simulink library "Enrg_conv_El_to_Mec_Bosch"  (R2016a)
settings: Solver=ode1  StartTime=0.0  StopTime=Inf  FixedStep=0.001  RelTol=1e-3
undefined symbols (not defined in the file): drvEmot_RefTqeMOT, FirstDrivenAxle_FirstDrivenAxleNoOfEmot, FMIKit, SecondDrivenAxle_SecondDrivenAxleNoOfEmot
libraries: Enrg_conv_El_to_Mec_Bosch x13, Electrical_converter x8
(part 1 of 5)
settings Model: Creator=SAHOPRA  LastModifiedBy=fschmi1
settings DataIOCC: LimitDataPoints=on  SaveFormat=Array
settings OptimizationCC: BlockReduction=off  OptimizeBlockIOStorage=off  BufferReuse=off  GlobalBufferReuse=off  ExpressionFolding=off  ExpressionDepthLimit=2147483647  LocalBlockOutputs=off
settings DebuggingCC: UnderspecifiedInitializationDetection=Classic  MergeDetectMultiDrivingBlocksExec=none  SolverPrmCheckMsg=warning  StateNameClashWarn=warning
settings HardwareCC: ProdBitPerPointer=32  ProdLargestAtomicFloat=None  ProdIntDivRoundTo=Undefined  ProdEndianess=Unspecified  ProdWordSize=32  ProdHWDeviceType=32-bit Generic
settings ModelReferenceCC: PropagateSignalLabelsOutOfModel=off
settings SFSimCC: SimUserSources="\"C:\\ORNOVNU\\01_DIVe\\drl_dev_hvlv_work\\ldDevProj\\case\\c000\\Content\\phys\\hvs\\Support\\FMIToolkit\\FMIKit-Simulink-2.9\\src\\FMU.cpp\" \"C:\\ORNOVNU\\01_DIVe\\drl_dev_hvlv_work\\ldDevProj\\case\\c000\\Content\\phys\\hvs\\Support\\FMIToolkit\\FMIKit-Simulink-2.9\\src\\FMU1.cpp\" \"C:\\ORNOVNU\\01_DIVe\\drl_dev_hvlv_work\\ldDevProj\\case\\c000\\Content\\phys\\hvs\\Support\\FMIToolkit\\FMIKit-Simulink-2.9\\src\\FMU2.cpp\" \"C:\\ORNOVNU\\01_DIVe\\drm_dev_hvlv_work\\Content\\phys\\hvs\\Support\\FMIToolkit\\FMIKit-Simulink-2.9\\src\\FMU.cpp\" \"C:\\ORNOVNU\\01_DIVe\\drm_dev_hvlv_work\\Content\\phys\\hvs\\Support\\FMIToolkit\\FMIKit-Simulink-2.9\\src\\FMU1.cpp\" \"C:\\ORNOVNU\\01_DIVe\\drm_dev_hvlv_work\\Content\\phys\\hvs\\Support\\FMIToolkit\\FMIKit-Simulink-2.9\\src\\FMU2.cpp\" \"C:\\ORNOVNU\\01_DIVe\\drm_dev_hvlv_work\\Content\\phys\\hvs\\detailed\\Support\\FMIToolkit\\FMIKit-Simulink-2.9\\src\\FMU.cpp\" \"C:\\ORNOVNU\\01_DIVe\\drm_dev_hvlv_work\\Content\\phys\\hvs\\detailed\\Support\\FMIToolkit\\FMIKit-Simulink-2.9\\src\\FMU1.cpp\" \"C:\\ORNOVNU\\01_DIVe\\drm_dev_hvlv_work\\Content\\phys\\hvs\\detailed\\Support\\FMIToolkit\\FMIKit-Simulink-2.9\\src\\FMU2.cpp\" \"Y:\\03_Tasks\\20210223_OrNu_HVSDive_BoschModelle\\02_WIP\\FMIKit-Simulink-2.9\\src\\FMU.cpp\" \"Y:\\03_Tasks\\20210223_OrNu_HVSDive_BoschModelle\\02_WIP\\FMIKit-Simulink-2.9\\src\\FMU1.cpp\" \"Y:\\03_Tasks\\20210223_OrNu_HVSDive_BoschModelle\\02_WIP\\FMIKit-Simulink-2.9\\src\\FMU2.cpp\" \"T:\\DIVe\\drm_dev_hvlv_work\\Content\\phys\\hvs\\detailed\\Support\\FMIToolkit\\FMIKit-Simulink-2.9\\src\\FMU.cpp\" \"T:\\DIVe\\drm_dev_hvlv_work\\Content\\phys\\hvs\\detailed\\Support\\FMIToolkit\\FMIKit-Simulink-2.9\\src\\FMU1.cpp\" \"T:\\DIVe\\drm_dev_hvlv_work\\Content\\phys\\hvs\\detailed\\Support\\FMIToolkit\\FMIKit-Simulink-2.9\\src\\FMU2.cpp\" \"c:\\ORNOVNU\\01_DIVe\\drm_dev_hvlv_work\\Content\\phys\\hvs\\detailed\\Support\\FMIToolkit\\FMIKit-Simulink-2.9\\src\\FMU.cpp\" \"c:\\ORNOVNU\\01_DIVe\\drm_dev_hvlv_work\\Content\\phys\\hvs\\detailed\\Support\\FMIToolkit\\FMIKit-Simulink-2.9\\src\\FMU1.cpp\" \"c:\\ORNOVNU\\01_DIVe\\drm_dev_hvlv_work\\Content\\phys\\hvs\\detailed\\Support\\FMIToolkit\\FMIKit-Simulink-2.9\\src\\FMU2.cpp\" \"D:\\01_DIVe\\drm_dev_hvlv_work\\Content\\phys\\hvs\\detailed\\Support\\FMIToolkit\\FMIKit-Simulink-2.9\\src\\FMU.cpp\" \"D:\\01_DIVe\\drm_dev_hvlv_work\\Content\\phys\\hvs\\detailed\\Support\\FMIToolkit\\FMIKit-Simulink-2.9\\src\\FMU1.cpp\" \"D:\\01_DIVe\\drm_dev_hvlv_work\\Content\\phys\\hvs\\detailed\\Support\\FMIToolkit\\FMIKit-Simulink-2.9\\src\\FMU2.cpp\" \"D:\\DIVe_Streams\\drm_dev_hvlv_work_1098\\Content\\phys\\hvs\\detailed\\Support\\FMIToolkit\\FMIKit-Simulink-2.9\\src\\FMU.cpp\" \"D:\\DIVe_Streams\\drm_dev_hvlv_work_1098\\Content\\phys\\hvs\\detailed\\Support\\FMIToolkit\\FMIKit-Simulink-2.9\\src\\FMU1.cpp\" \"D:\\DIVe_Streams\\drm_dev_hvlv_work_1098\\Content\\phys\\hvs\\detailed\\Support\\FMIToolkit\\FMIKit-Simulink-2.9\\src\\FMU2.cpp\""  SimUserIncludeDirs="\"C:\\ORNOVNU\\01_DIVe\\drl_dev_hvlv_work\\ldDevProj\\case\\c000\\Content\\phys\\hvs\\Support\\FMIToolkit\\FMIKit-Simulink-2.9\\include\" \"C:\\ORNOVNU\\01_DIVe\\drm_dev_hvlv_work\\Content\\phys\\hvs\\Support\\FMIToolkit\\FMIKit-Simulink-2.9\\include\" \"C:\\ORNOVNU\\01_DIVe\\drm_dev_hvlv_work\\Content\\phys\\hvs\\detailed\\Support\\FMIToolkit\\FMIKit-Simulink-2.9\\include\" \"Y:\\03_Tasks\\20210223_OrNu_HVSDive_BoschModelle\\02_WIP\\FMIKit-Simulink-2.9\\include\" \"T:\\DIVe\\drm_dev_hvlv_work\\Content\\phys\\hvs\\detailed\\Support\\FMIToolkit\\FMIKit-Simulink-2.9\\include\" \"c:\\ORNOVNU\\01_DIVe\\drm_dev_hvlv_work\\Content\\phys\\hvs\\detailed\\Support\\FMIToolkit\\FMIKit-Simulink-2.9\\include\" \"D:\\01_DIVe\\drm_dev_hvlv_work\\Content\\phys\\hvs\\detailed\\Support\\FMIToolkit\\FMIKit-Simulink-2.9\\include\" \"D:\\DIVe_Streams\\drm_dev_hvlv_work_1098\\Content\\phys\\hvs\\detailed\\Support\\FMIToolkit\\FMIKit-Simulink-2.9\\include\""
settings RTWCC: SystemTargetFile=rti1005.tlc  MakeCommand=make_rti  TemplateMakefile=rti1005.tmf  Description=dSPACE DS1005 Hardware Platform  CustomInclude="\"C:\\ORNOVNU\\01_DIVe\\drl_dev_hvlv_work\\ldDevProj\\case\\c000\\Content\\phys\\hvs\\Support\\FMIToolkit\\FMIKit-Simulink-2.9\\include\" \"C:\\ORNOVNU\\01_DIVe\\drm_dev_hvlv_work\\Content\\phys\\hvs\\Support\\FMIToolkit\\FMIKit-Simulink-2.9\\include\" \"C:\\ORNOVNU\\01_DIVe\\drm_dev_hvlv_work\\Content\\phys\\hvs\\detailed\\Support\\FMIToolkit\\FMIKit-Simulink-2.9\\include\" \"Y:\\03_Tasks\\20210223_OrNu_HVSDive_BoschModelle\\02_WIP\\FMIKit-Simulink-2.9\\include\" \"T:\\DIVe\\drm_dev_hvlv_work\\Content\\phys\\hvs\\detailed\\Support\\FMIToolkit\\FMIKit-Simulink-2.9\\include\" \"c:\\ORNOVNU\\01_DIVe\\drm_dev_hvlv_work\\Content\\phys\\hvs\\detailed\\Support\\FMIToolkit\\FMIKit-Simulink-2.9\\include\" \"D:\\01_DIVe\\drm_dev_hvlv_work\\Content\\phys\\hvs\\detailed\\Support\\FMIToolkit\\FMIKit-Simulink-2.9\\include\" \"D:\\DIVe_Streams\\drm_dev_hvlv_work_1098\\Content\\phys\\hvs\\detailed\\Support\\FMIToolkit\\FMIKit-Simulink-2.9\\include\""  CustomSource="\"C:\\ORNOVNU\\01_DIVe\\drl_dev_hvlv_work\\ldDevProj\\case\\c000\\Content\\phys\\hvs\\Support\\FMIToolkit\\FMIKit-Simulink-2.9\\src\\FMU.cpp\" \"C:\\ORNOVNU\\01_DIVe\\drl_dev_hvlv_work\\ldDevProj\\case\\c000\\Content\\phys\\hvs\\Support\\FMIToolkit\\FMIKit-Simulink-2.9\\src\\FMU1.cpp\" \"C:\\ORNOVNU\\01_DIVe\\drl_dev_hvlv_work\\ldDevProj\\case\\c000\\Content\\phys\\hvs\\Support\\FMIToolkit\\FMIKit-Simulink-2.9\\src\\FMU2.cpp\" \"C:\\ORNOVNU\\01_DIVe\\drm_dev_hvlv_work\\Content\\phys\\hvs\\Support\\FMIToolkit\\FMIKit-Simulink-2.9\\src\\FMU.cpp\" \"C:\\ORNOVNU\\01_DIVe\\drm_dev_hvlv_work\\Content\\phys\\hvs\\Support\\FMIToolkit\\FMIKit-Simulink-2.9\\src\\FMU1.cpp\" \"C:\\ORNOVNU\\01_DIVe\\drm_dev_hvlv_work\\Content\\phys\\hvs\\Support\\FMIToolkit\\FMIKit-Simulink-2.9\\src\\FMU2.cpp\" \"C:\\ORNOVNU\\01_DIVe\\drm_dev_hvlv_work\\Content\\phys\\hvs\\detailed\\Support\\FMIToolkit\\FMIKit-Simulink-2.9\\src\\FMU.cpp\" \"C:\\ORNOVNU\\01_DIVe\\drm_dev_hvlv_work\\Content\\phys\\hvs\\detailed\\Support\\FMIToolkit\\FMIKit-Simulink-2.9\\src\\FMU1.cpp\" \"C:\\ORNOVNU\\01_DIVe\\drm_dev_hvlv_work\\Content\\phys\\hvs\\detailed\\Support\\FMIToolkit\\FMIKit-Simulink-2.9\\src\\FMU2.cpp\" \"Y:\\03_Tasks\\20210223_OrNu_HVSDive_BoschModelle\\02_WIP\\FMIKit-Simulink-2.9\\src\\FMU.cpp\" \"Y:\\03_Tasks\\20210223_OrNu_HVSDive_BoschModelle\\02_WIP\\FMIKit-Simulink-2.9\\src\\FMU1.cpp\" \"Y:\\03_Tasks\\20210223_OrNu_HVSDive_BoschModelle\\02_WIP\\FMIKit-Simulink-2.9\\src\\FMU2.cpp\" \"T:\\DIVe\\drm_dev_hvlv_work\\Content\\phys\\hvs\\detailed\\Support\\FMIToolkit\\FMIKit-Simulink-2.9\\src\\FMU.cpp\" \"T:\\DIVe\\drm_dev_hvlv_work\\Content\\phys\\hvs\\detailed\\Support\\FMIToolkit\\FMIKit-Simulink-2.9\\src\\FMU1.cpp\" \"T:\\DIVe\\drm_dev_hvlv_work\\Content\\phys\\hvs\\detailed\\Support\\FMIToolkit\\FMIKit-Simulink-2.9\\src\\FMU2.cpp\" \"c:\\ORNOVNU\\01_DIVe\\drm_dev_hvlv_work\\Content\\phys\\hvs\\detailed\\Support\\FMIToolkit\\FMIKit-Simulink-2.9\\src\\FMU.cpp\" \"c:\\ORNOVNU\\01_DIVe\\drm_dev_hvlv_work\\Content\\phys\\hvs\\detailed\\Support\\FMIToolkit\\FMIKit-Simulink-2.9\\src\\FMU1.cpp\" \"c:\\ORNOVNU\\01_DIVe\\drm_dev_hvlv_work\\Content\\phys\\hvs\\detailed\\Support\\FMIToolkit\\FMIKit-Simulink-2.9\\src\\FMU2.cpp\" \"D:\\01_DIVe\\drm_dev_hvlv_work\\Content\\phys\\hvs\\detailed\\Support\\FMIToolkit\\FMIKit-Simulink-2.9\\src\\FMU.cpp\" \"D:\\01_DIVe\\drm_dev_hvlv_work\\Content\\phys\\hvs\\detailed\\Support\\FMIToolkit\\FMIKit-Simulink-2.9\\src\\FMU1.cpp\" \"D:\\01_DIVe\\drm_dev_hvlv_work\\Content\\phys\\hvs\\detailed\\Support\\FMIToolkit\\FMIKit-Simulink-2.9\\src\\FMU2.cpp\" \"D:\\DIVe_Streams\\drm_dev_hvlv_work_1098\\Content\\phys\\hvs\\detailed\\Support\\FMIToolkit\\FMIKit-Simulink-2.9\\src\\FMU.cpp\" \"D:\\DIVe_Streams\\drm_dev_hvlv_work_1098\\Content\\phys\\hvs\\detailed\\Support\\FMIToolkit\\FMIKit-Simulink-2.9\\src\\FMU1.cpp\" \"D:\\DIVe_Streams\\drm_dev_hvlv_work_1098\\Content\\phys\\hvs\\detailed\\Support\\FMIToolkit\\FMIKit-Simulink-2.9\\src\\FMU2.cpp\""
settings STFCustomTargetCC: ModelReferenceCompliant=off  GeneratePreprocessorConditionals=Disable all  CombineOutputUpdateFcns=on  MatFileLogging=on  CPPClassGenCompliant=on  GRTInterface=off  SystemTargetFile=rti1005.tlc
settings GRTTargetCC: ModelReferenceCompliant=off  ParMdlRefBuildCompliant=off  CompOptLevelCompliant=off  ConcurrentExecutionCompliant=off  UseToolchainInfoCompliant=off
settings ConfigComp: CovModelRefEnable=Off

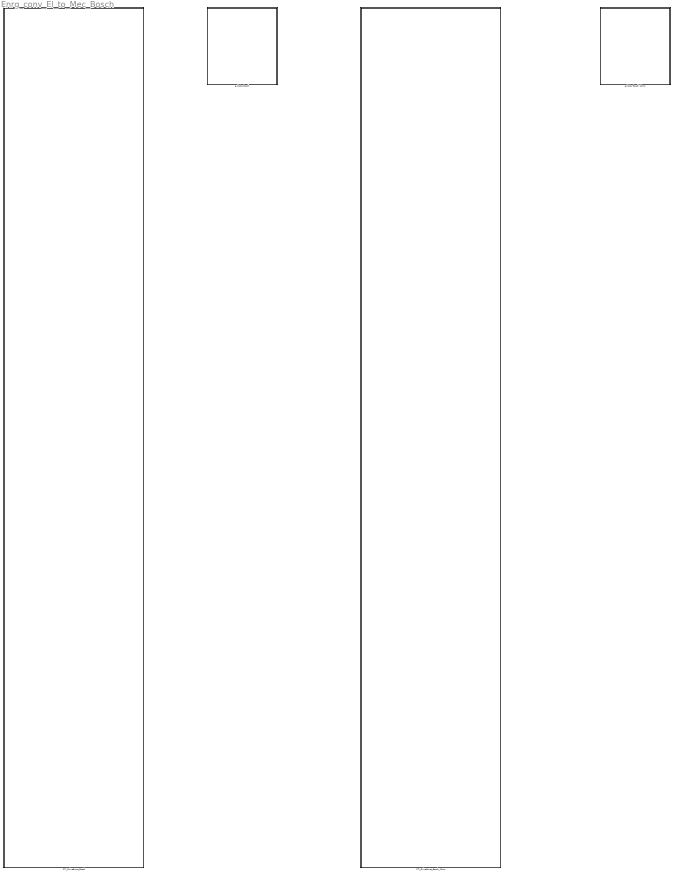
== system Enrg_conv_El_to_Mec_Bosch ==
  PTI_DriveEmot_Bosch : Subsystem  TreatAsAtomicUnit=on  SystemSampleTime=0.1
  PTI_DriveEmot_Bosch_10ms : Subsystem  TreatAsAtomicUnit=on  SystemSampleTime=0.01
  e-Motor Bosch : Subsystem  mask(MapModule){}
  e-Motor Bosch 10ms : Subsystem  mask(MapModule){}

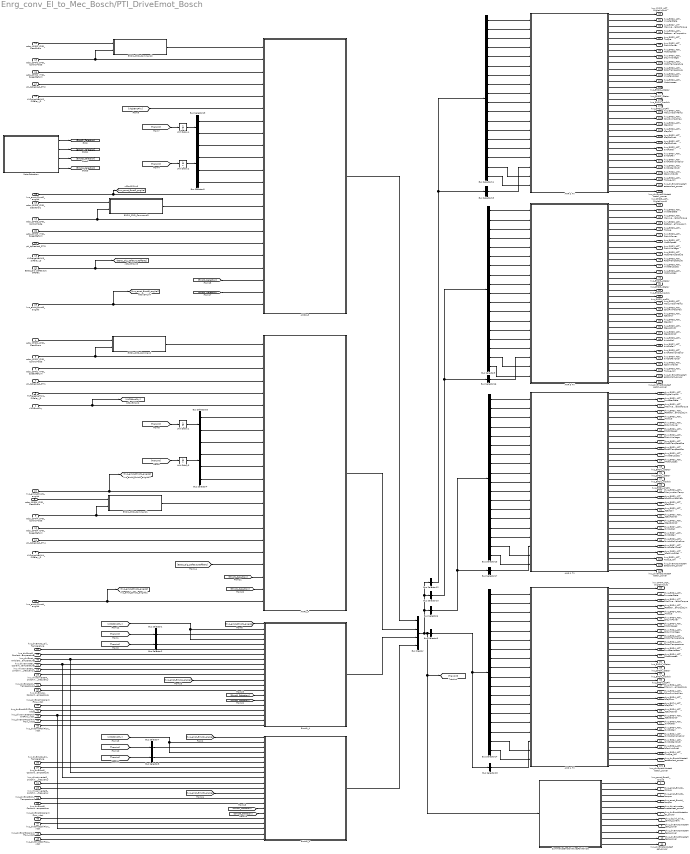
== system Enrg_conv_El_to_Mec_Bosch/PTI_DriveEmot_Bosch ==
  vltZkBmsPhy : Inport
  HVFreigabeHW1_SiRelay_D : Inport  Port=2
  HVFreigabeHW4_SiRelay_D : Inport  Port=3
  edcu_EMD1_CMD_ClearErrors : Inport  Port=4
  edcu_EMD1_CMD_ControlMode : Inport  Port=5
  edcu_EMD1_CMD_SpeedRefLim : Inport  Port=6
  pti_tqDesired_PTI1 : Inport  Description=[Nm]  Port=7
      settings: AttributesFormatString=%<Description>
  edcu_EMD4_CMD_ClearErrors : Inport  Port=8
  edcu_EMD4_CMD_ControlMode : Inport  Port=9
  edcu_EMD4_CMD_SpeedRefLim : Inport  Port=10
  pti_tqDesired_PTI4 : Inport  Description=[Nm]  Port=11
      settings: AttributesFormatString=%<Description>
  HVFreigabeHW2_SiRelay_D : Inport  Port=12
  HVFreigabeHW3_SiRelay_D : Inport  Port=13
  edcu_EMD2_CMD_ClearErrors : Inport  Port=14
  edcu_EMD2_CMD_ControlMode : Inport  Port=15
  edcu_EMD2_CMD_SpeedRefLim : Inport  Port=16
  pti_tqDesired_PTI2 : Inport  Description=[Nm]  Port=17
      settings: AttributesFormatString=%<Description>
  edcu_EMD3_CMD_ClearErrors : Inport  Port=18
  edcu_EMD3_CMD_ControlMode : Inport  Port=19
  edcu_EMD3_CMD_SpeedRefLim : Inport  Port=20
  pti_tqDesired_PTI3 : Inport  Description=[Nm]  Port=21
      settings: AttributesFormatString=%<Description>
  EDCU_Dig_SafetyCutOffDG1 : Inport  Port=22
  hvs_driveInverter1_switching_frequency : Inport  Port=23
  hvs_driveInverter2_switching_frequency : Inport  Port=24
  hvs_driveInverter3_switching_frequency : Inport  Port=25
  hvs_driveInverter4_switching_frequency : Inport  Port=26
  hvs_emot_Emot1_angVel : Inport  Port=27
  hvs_emot_Emot2_angVel : Inport  Port=28
  hvs_emot_Emot3_angVel : Inport  Port=29
  hvs_emot_Emot4_angVel : Inport  Port=30
  hvs_driveInverter_coolant_temperature : Inport  Port=31
  hvs_drvEmot1_Oil_Temperature : Inport  Port=32
  hvs_drvEmot1_Coolant_Temperature : Inport  Port=33
  hvs_drvEmot4Oil_Temperature : Inport  Port=34
  hvs_drvEmot4_Coolant_Temperature : Inport  Port=35
  hvs_drvEmot2_Oil_Temperature : Inport  Port=36
  hvs_drvEmot2_Coolant_Temperature : Inport  Port=37
  hvs_drvEmot3Oil_Temperature : Inport  Port=38
  hvs_drvEmot3_Coolant_Temperature : Inport  Port=39
  hvs_drvEmot_Ambient_Temperature : Inport  Port=40
  hvs_drvEmot1CoolantFlow_vdot : Inport  Port=41
  hvs_drvEmot1OilFlow_vdot : Inport  Port=42
  hvs_driveInverterCoolantFlow_vdot : Inport  Port=43
  hvs_drvEmot4CoolantFlow_vdot : Inport  Port=44
  hvs_drvEmot4OilFlow_vdot : Inport  Port=45
  hvs_drvEmot2CoolantFlow_vdot : Inport  Port=46
  hvs_drvEmot2OilFlow_vdot : Inport  Port=47
  hvs_drvEmot3CoolantFlow_vdot : Inport  Port=48
  hvs_drvEmot3OilFlow_vdot : Inport  Port=49
  AWR 1 TX : Subsystem
  AWR 2 TX : Subsystem
  AWR 3 TX : Subsystem
  AWR 4 TX : Subsystem
  AWR1_4 : Subsystem
  AWR2_3 : Subsystem
  Bus Selector11 : BusSelector  OutputSignals=EMD2_ACT_DcLinkVoltage,EMD_ACT_DigitalInput1,EMD_ACT_MaximumAvailableTorque,EMD_ACT_DcLinkPower,EMD_ACT_MotorSpeed,EMD_ACT_MotorTorque,EMD_ACT_InverterState,EMD_ACT_ReferenceTorqueLimited,drvEmot_T_Stator,drvEmot_T_Rotor,Inv_Ploss,mot_Ploss,uStator,iStator,modIdx,cosPhi,wasteHeat_coolant,wasteHeat_oil
  Bus Selector13 : BusSelector  OutputSignals=EMD1_ACT_DcLinkVoltage,EMD_ACT_DigitalInput1,EMD_ACT_MaximumAvailableTorque,EMD_ACT_DcLinkPower,EMD_ACT_MotorSpeed,EMD_ACT_MotorTorque,EMD_ACT_InverterState,EMD_ACT_ReferenceTorqueLimited,drvEmot_T_Stator,drvEmot_T_Rotor,Inv_Ploss,mot_Ploss,uStator,iStator,modIdx,cosPhi,wasteHeat_coolant,wasteHeat_oil
  Bus Selector14 : BusSelector  OutputSignals=EMD4_ACT_DcLinkVoltage,EMD_ACT_DigitalInput1,EMD_ACT_MaximumAvailableTorque,EMD_ACT_DcLinkPower,EMD_ACT_MotorSpeed,EMD_ACT_MotorTorque,EMD_ACT_InverterState,EMD_ACT_ReferenceTorqueLimited,drvEmot_T_Stator,drvEmot_T_Rotor,Inv_Ploss,mot_Ploss,uStator,iStator,modIdx,cosPhi,wasteHeat_coolant,wasteHeat_oil
  Bus Selector{15..18} (4 alike) : BusSelector  OutputSignals=driveInverter_Temperatures  OutputAsBus=on
  Bus Selector9 : BusSelector  OutputSignals=EMD3_ACT_DcLinkVoltage,EMD_ACT_DigitalInput1,EMD_ACT_MaximumAvailableTorque,EMD_ACT_DcLinkPower,EMD_ACT_MotorSpeed,EMD_ACT_MotorTorque,EMD_ACT_InverterState,EMD_ACT_ReferenceTorqueLimited,drvEmot_T_Stator,drvEmot_T_Rotor,Inv_Ploss,mot_Ploss,uStator,iStator,modIdx,cosPhi,wasteHeat_oil,wasteHeat_coolant
  Bus Creator : BusCreator  Inputs=4
  Bus Selector1 : BusSelector  OutputSignals=awr1_4B.awr1B.trqEmotDesPhy
  Bus Selector10 : BusSelector  OutputSignals=awr2_3B.awr3B.EMD3_ACT_DcLinkVoltage,awr2_3B.awr3B.EMD_ACT_DigitalInput1,awr2_3B.awr3B.EMD_ACT_MaximumAvailableTorque,awr2_3B.awr3B.EMD_ACT_DcLinkPower,awr2_3B.awr3B.EMD_ACT_MotorSpeed,awr2_3B.awr3B.EMD_ACT_MotorTorque,awr2_3B.awr3B.EMD_ACT_InverterState,awr2_3B.awr3B.EMD_ACT_ReferenceTorqueLimited,awr2_3B.awr3B.trqEmotDesPhy,emot2_3B.emot3B.driveInverter_Temperatures,emot2_3B.emot3B.drvEmot_T_Stator,emot2_3B.emot3B.drvEmot_T_Rotor,emot2_3B.emot3B.Inv_Ploss,emot2_3B.emot3B.mot_Ploss,emot2_3B.emot3B.uStator,emot2_3B.emot3B.iStator,emot2_3B.emot3B.modIdx,emot2_3B.emot3B.cosPhi,emot2_3B.emot3B.wasteHeat_coolant,emot2_3B.emot3B.wasteHeat_oil  OutputAsBus=on
  Bus Selector12 : BusSelector  OutputSignals=awr2_3B.awr2B.EMD2_ACT_DcLinkVoltage,awr2_3B.awr2B.EMD_ACT_DigitalInput1,awr2_3B.awr2B.EMD_ACT_MaximumAvailableTorque,awr2_3B.awr2B.EMD_ACT_DcLinkPower,awr2_3B.awr2B.EMD_ACT_MotorSpeed,awr2_3B.awr2B.EMD_ACT_MotorTorque,awr2_3B.awr2B.EMD_ACT_InverterState,awr2_3B.awr2B.EMD_ACT_ReferenceTorqueLimited,awr2_3B.awr2B.trqEmotDesPhy,emot2_3B.emot2B.driveInverter_Temperatures,emot2_3B.emot2B.drvEmot_T_Stator,emot2_3B.emot2B.drvEmot_T_Rotor,emot2_3B.emot2B.Inv_Ploss,emot2_3B.emot2B.mot_Ploss,emot2_3B.emot2B.uStator,emot2_3B.emot2B.iStator,emot2_3B.emot2B.modIdx,emot2_3B.emot2B.cosPhi,emot2_3B.emot2B.wasteHeat_coolant,emot2_3B.emot2B.wasteHeat_oil  OutputAsBus=on
  Bus Selector19 : BusSelector  OutputSignals=emot2_3B.emot2B.trqEmotPhy,emot2_3B.emot3B.trqEmotPhy
  Bus Selector2 : BusSelector  OutputSignals=awr1_4B.awr4B.trqEmotDesPhy
  Bus Selector20 : BusSelector  OutputSignals=emot1_4B.emot1B.trqEmotPhy,emot1_4B.emot4B.trqEmotPhy
  Bus Selector3 : BusSelector  OutputSignals=emot2_3B.emot2B.pwrEmotPhy,emot2_3B.emot3B.pwrEmotPhy,emot2_3B.emot2B.trqEmotMax,emot2_3B.emot3B.trqEmotMax
  Bus Selector4 : BusSelector  OutputSignals=emot1_4B.emot1B.pwrEmotPhy,emot1_4B.emot4B.pwrEmotPhy,emot1_4B.emot1B.trqEmotMax,emot1_4B.emot4B.trqEmotMax
  Bus Selector5 : BusSelector  OutputSignals=awr1_4B.awr4B.EMD4_ACT_DcLinkVoltage,awr1_4B.awr4B.EMD_ACT_DigitalInput1,awr1_4B.awr4B.EMD_ACT_MaximumAvailableTorque,awr1_4B.awr4B.EMD_ACT_DcLinkPower,awr1_4B.awr4B.EMD_ACT_MotorSpeed,awr1_4B.awr4B.EMD_ACT_MotorTorque,awr1_4B.awr4B.EMD_ACT_InverterState,awr1_4B.awr4B.EMD_ACT_ReferenceTorqueLimited,awr1_4B.awr4B.trqEmotDesPhy,emot1_4B.emot4B.driveInverter_Temperatures,emot1_4B.emot4B.drvEmot_T_Stator,emot1_4B.emot4B.drvEmot_T_Rotor,emot1_4B.emot4B.Inv_Ploss,emot1_4B.emot4B.mot_Ploss,emot1_4B.emot4B.uStator,emot1_4B.emot4B.iStator,emot1_4B.emot4B.modIdx,emot1_4B.emot4B.cosPhi,emot1_4B.emot4B.wasteHeat_coolant,emot1_4B.emot4B.wasteHeat_oil  OutputAsBus=on
  Bus Selector6 : BusSelector  OutputSignals=awr1_4B.awr1B.EMD1_ACT_DcLinkVoltage,awr1_4B.awr1B.EMD_ACT_DigitalInput1,awr1_4B.awr1B.EMD_ACT_MaximumAvailableTorque,awr1_4B.awr1B.EMD_ACT_DcLinkPower,awr1_4B.awr1B.EMD_ACT_MotorSpeed,awr1_4B.awr1B.EMD_ACT_MotorTorque,awr1_4B.awr1B.EMD_ACT_InverterState,awr1_4B.awr1B.EMD_ACT_ReferenceTorqueLimited,awr1_4B.awr1B.trqEmotDesPhy,emot1_4B.emot1B.driveInverter_Temperatures,emot1_4B.emot1B.drvEmot_T_Stator,emot1_4B.emot1B.drvEmot_T_Rotor,emot1_4B.emot1B.Inv_Ploss,emot1_4B.emot1B.mot_Ploss,emot1_4B.emot1B.uStator,emot1_4B.emot1B.iStator,emot1_4B.emot1B.modIdx,emot1_4B.emot1B.cosPhi,emot1_4B.emot1B.wasteHeat_coolant,emot1_4B.emot1B.wasteHeat_oil  OutputAsBus=on
  Bus Selector7 : BusSelector  OutputSignals=awr2_3B.awr2B.trqEmotDesPhy
  Bus Selector8 : BusSelector  OutputSignals=awr2_3B.awr3B.trqEmotDesPhy
  EMD1_CMD_Command : Subsystem
  EMD1_CMD_Command1 : Subsystem
  EMD1_CMD_Command2 : Subsystem
  EMD1_CMD_Command3 : Subsystem
  Emot1_4 : Subsystem
  Emot2_3 : Subsystem
  MotorSelection : Subsystem
  SummarizeEmotorValuesForVehicle : Subsystem  TreatAsAtomicUnit=on
  Unit Delay{1..4} (4 alike) : UnitDelay  SampleTime=-1
  hvs_dcLink_drive_emot_current : Outport
  hvs_emot_Emot1_torque : Outport  Port=2
  hvs_emot_Emot2_torque : Outport  Port=3
  hvs_emot_Emot3_torque : Outport  Port=4
  hvs_emot_Emot4_torque : Outport  Port=5
  hvs_driveInverter_wasteHeat_power : Outport  Port=6
  hvs_drvEmotWasteHeat_power : Outport  Port=7
  hvs_drvEmot1WasteHeat_power : Outport  Port=8
  hvs_drvEmot2WasteHeat_power : Outport  Port=9
  hvs_drvEmot3WasteHeat_power : Outport  Port=10
  hvs_drvEmot4WasteHeat_power : Outport  Port=11
  hvs_EMD1_ACT_DigitalInput1 : Outport  Port=12
  hvs_EMD1_ACT_InverterState : Outport  Port=13
  hvs_EMD1_ACT_MaxAvailableTorque : Outport  Port=14
  hvs_EMD1_ACT_ReferenceTorqueLim : Outport  Port=15
  hvs_EMD1_ACT_Torque : Outport  Port=16
  hvs_EMD1_ACT_DcLinkPower : Outport  Port=17
  hvs_EMD1_ACT_MotorSpeed : Outport  Port=18
  hvs_EMD1_ACT_DcLinkVoltage : Outport  Port=19
  hvs_EMD1_ACT_MaxJunctionTemp : Outport  Port=20
  hvs_EMD1_ACT_MotorTemperature : Outport  Port=21
  hvs_EMD1_ACT_RotorTemperature : Outport  Port=22
  hvs_EMD1_ACT_InverterLosses : Outport  Port=23
  hvs_EMD1_ACT_MotorLosses : Outport  Port=24
  hvs_EMD1_uStator : Outport  Port=25
  hvs_EMD1_iStator : Outport  Port=26
  hvs_EMD1_modIdx : Outport  Port=27
  hvs_EMD1_cosPhi : Outport  Port=28
  hvs_EMD1_ACT_tSnsrPwrModlMax : Outport  Port=29
  hvs_EMD1_ACT_tCapSnsr : Outport  Port=30
  hvs_EMD1_ACT_tCapCoil : Outport  Port=31
  hvs_EMD1_ACT_tCapAcCnctr : Outport  Port=32
  hvs_EMD1_ACT_tCapDcCnctr : Outport  Port=33
  hvs_EMD1_ACT_tIvtrAcRail : Outport  Port=34
  hvs_EMD1_ACT_tIvtrDcRail : Outport  Port=35
  hvs_EMD1_ACT_tIvtrAcRailIphaSnsr : Outport  Port=36
  hvs_EMD1_ACT_tIvtrDcRailCnctr : Outport  Port=37
  hvs_EMD1_ACT_tCoolIvtrOuttk : Outport  Port=38
  hvs_EMD4_ACT_DigitalInput1 : Outport  Port=39
  hvs_EMD4_ACT_InverterState : Outport  Port=40
  hvs_EMD4_ACT_MaxAvailableTorque : Outport  Port=41
  hvs_EMD4_ACT_ReferenceTorqueLim : Outport  Port=42
  hvs_EMD4_ACT_Torque : Outport  Port=43
  hvs_EMD4_ACT_DcLinkPower : Outport  Port=44
  hvs_EMD4_ACT_MotorSpeed : Outport  Port=45
  hvs_EMD4_ACT_DcLinkVoltage : Outport  Port=46
  hvs_EMD4_ACT_MaxJunctionTemperature : Outport  Port=47
  hvs_EMD4_ACT_MotorTemperature : Outport  Port=48
  hvs_EMD4_ACT_RotorTemperature : Outport  Port=49
  hvs_EMD4_ACT_InverterLosses : Outport  Port=50
  hvs_EMD4_ACT_MotorLosses : Outport  Port=51
  hvs_EMD4_uStator : Outport  Port=52
  hvs_EMD4_iStator : Outport  Port=53
  hvs_EMD4_modIdx : Outport  Port=54
  hvs_EMD4_cosPhi : Outport  Port=55
  hvs_EMD4_ACT_tSnsrPwrModlMax : Outport  Port=56
  hvs_EMD4_ACT_tCapSnsr : Outport  Port=57
  hvs_EMD4_ACT_tCapCoil : Outport  Port=58
  hvs_EMD4_ACT_tCapAcCnctr : Outport  Port=59
  hvs_EMD4_ACT_tCapDcCnctr : Outport  Port=60
  hvs_EMD4_ACT_tIvtrAcRail : Outport  Port=61
  hvs_EMD4_ACT_tIvtrDcRail : Outport  Port=62
  hvs_EMD4_ACT_tIvtrAcRailIphaSnsr : Outport  Port=63
  hvs_EMD4_ACT_tIvtrDcRailCnctr : Outport  Port=64
  hvs_EMD4_ACT_tCoolIvtrOuttk : Outport  Port=65
  hvs_EMD3_ACT_DigitalInput1 : Outport  Port=66
  hvs_EMD3_ACT_InverterState : Outport  Port=67
  hvs_EMD3_ACT_MaxAvailableTorque : Outport  Port=68
  hvs_EMD3_ACT_ReferenceTorqueLim : Outport  Port=69
  hvs_EMD3_ACT_Torque : Outport  Port=70
  hvs_EMD3_ACT_DcLinkPower : Outport  Port=71
  hvs_EMD3_ACT_MotorSpeed : Outport  Port=72
  hvs_EMD3_ACT_DcLinkVoltage : Outport  Port=73
  hvs_EMD3_ACT_MaxJunctionTemp : Outport  Port=74
  hvs_EMD3_ACT_MotorTemperature : Outport  Port=75
  hvs_EMD3_ACT_RotorTemperature : Outport  Port=76
  hvs_EMD3_ACT_InverterLosses : Outport  Port=77
  hvs_EMD3_ACT_MotorLosses : Outport  Port=78
  hvs_EMD3_uStator : Outport  Port=79
  hvs_EMD3_iStator : Outport  Port=80
  hvs_EMD3_modIdx : Outport  Port=81
  hvs_EMD3_cosPhi : Outport  Port=82
  hvs_EMD3_ACT_tSnsrPwrModlMax : Outport  Port=83
  hvs_EMD3_ACT_tCapSnsr : Outport  Port=84
  hvs_EMD3_ACT_tCapCoil : Outport  Port=85
  hvs_EMD3_ACT_tCapAcCnctr : Outport  Port=86
  hvs_EMD3_ACT_tCapDcCnctr : Outport  Port=87
  hvs_EMD3_ACT_tIvtrAcRail : Outport  Port=88
  hvs_EMD3_ACT_tIvtrDcRail : Outport  Port=89
  hvs_EMD3_ACT_tIvtrAcRailIphaSnsr : Outport  Port=90
  hvs_EMD3_ACT_tIvtrDcRailCnctr : Outport  Port=91
  hvs_EMD3_ACT_tCoolIvtrOuttk : Outport  Port=92
  hvs_EMD2_ACT_DigitalInput1 : Outport  Port=93
  hvs_EMD2_ACT_InverterState : Outport  Port=94
  hvs_EMD2_ACT_MaxAvailableTorque : Outport  Port=95
  hvs_EMD2_ACT_ReferenceTorqueLim : Outport  Port=96
  hvs_EMD2_ACT_Torque : Outport  Port=97
  hvs_EMD2_ACT_DcLinkPower : Outport  Port=98
  hvs_EMD2_ACT_MotorSpeed : Outport  Port=99
  hvs_EMD2_ACT_DcLinkVoltage : Outport  Port=100
  hvs_EMD2_ACT_MaxJunctionTemp : Outport  Port=101
  hvs_EMD2_ACT_MotorTemperature : Outport  Port=102
  hvs_EMD2_ACT_RotorTemperature : Outport  Port=103
  hvs_EMD2_ACT_InverterLosses : Outport  Port=104
  hvs_EMD2_ACT_MotorLosses : Outport  Port=105
  hvs_EMD2_uStator : Outport  Port=106
  hvs_EMD2_iStator : Outport  Port=107
  hvs_EMD2_modIdx : Outport  Port=108
  hvs_EMD2_cosPhi : Outport  Port=109
  hvs_EMD2_ACT_tSnsrPwrModlMax : Outport  Port=110
  hvs_EMD2_ACT_tCapSnsr : Outport  Port=111
  hvs_EMD2_ACT_tCapCoil : Outport  Port=112
  hvs_EMD2_ACT_tCapAcCnctr : Outport  Port=113
  hvs_EMD2_ACT_tCapDcCnctr : Outport  Port=114
  hvs_EMD2_ACT_tIvtrAcRail : Outport  Port=115
  hvs_EMD2_ACT_tIvtrDcRail : Outport  Port=116
  hvs_EMD2_ACT_tIvtrAcRailIphaSnsr : Outport  Port=117
  hvs_EMD2_ACT_tIvtrDcRailCnctr : Outport  Port=118
  hvs_EMD2_ACT_tCoolIvtrOuttk : Outport  Port=119
  hvs_EMD2_ACT_Torque_Nm : Outport  Port=120
  hvs_EMD3_ACT_Torque_Nm : Outport  Port=121
  hvs_EMD1_ACT_Torque_Nm : Outport  Port=122
  hvs_EMD4_ACT_Torque_Nm : Outport  Port=123
  hvs_drvEmot2WasteHeatcoolant_power : Outport  Port=124
  hvs_drvEmot2WasteHeatoil_power : Outport  Port=125
  hvs_drvEmot3WasteHeatcoolant_power : Outport  Port=126
  hvs_drvEmot3WasteHeatoil_power : Outport  Port=127
  hvs_drvEmot1WasteHeatcoolant_power : Outport  Port=128
  hvs_drvEmot1WasteHeatoil_power : Outport  Port=129
  hvs_drvEmot4WasteHeatcoolant_power : Outport  Port=130
  hvs_drvEmot4WasteHeatoil_power : Outport  Port=131
  wires:
  Bus Selector20/2 -> AWR1_4/8(trqEmot4Phy)  "<trqEmotPhy>"
  Bus Selector20/1 -> AWR1_4/7(trqEmot1Phy)  "<trqEmotPhy>"
  [TransInt] -> Unit Delay1/1
  Bus Selector19/2 -> AWR2_3/8(trqEmot3Phy)  "<trqEmotPhy>"
  Bus Selector19/1 -> AWR2_3/7(trqEmot2Phy)  "<trqEmotPhy>"
  [TransInt] -> Unit Delay4/1
  hvs_driveInverter_coolant_temperature/1 -> Emot2_3/9(inv_coolant_temperature), Emot1_4/9(inv_coolant_temperature)
  hvs_drvEmot1_Oil_Temperature/1 -> Emot1_4/6(drvEmot1_Oil_Temperature)
  Bus Selector5/1 -> Bus Selector14/1, Bus Selector18/1  "TransInt"
  edcu_EMD1_CMD_ControlMode/1 -> EMD1_CMD_Command/2(EMD1_CMD_MotorControlMode), AWR1_4/2(EMD1_CMD_MotorControlMode)
  edcu_EMD1_CMD_ClearErrors/1 -> EMD1_CMD_Command/1(EMD1_CMD_ClearErrors)
  vltZkBmsPhy/1 -> [vltZkBmsPhy], AWR1_4/6(vltZkBmsPhy)
  hvs_emot_Emot1_angVel/1 -> [hvs_emot_Emot1_angVel], AWR1_4/13(hvs_emot_Emot1_angVel)
  edcu_EMD4_CMD_ControlMode/1 -> EMD1_CMD_Command1/2(EMD1_CMD_MotorControlMode), AWR1_4/15(EMD4_CMD_MotorControlMode)
  edcu_EMD4_CMD_ClearErrors/1 -> EMD1_CMD_Command1/1(EMD1_CMD_ClearErrors)
  Bus Creator/1 -> [TransInt], SummarizeEmotorValuesForVehicle/1(MultiBus_Emot_Inv_1_4), Bus Selector5/1, Bus Selector12/1, Bus Selector10/1, Bus Selector6/1  "TransInt"
  Bus Selector6/1 -> Bus Selector13/1, Bus Selector17/1  "TransInt"
  SummarizeEmotorValuesForVehicle/1(hvs_emot_Emot1_torque) -> hvs_emot_Emot1_torque/1
  SummarizeEmotorValuesForVehicle/7(hvs_dcLink_drive_emot_current) -> hvs_dcLink_drive_emot_current/1
  SummarizeEmotorValuesForVehicle/6(hvs_drvEmotWasteHeat_power) -> hvs_drvEmotWasteHeat_power/1
  SummarizeEmotorValuesForVehicle/5(hvs_driveInverter_wasteHeat_power) -> hvs_driveInverter_wasteHeat_power/1
  [TransInt] -> Bus Selector1/1
  [TransInt] -> Bus Selector2/1
  [TransInt] -> Unit Delay3/1
  Unit Delay3/1 -> Bus Selector4/1
  EMD1_CMD_Command/1(Out_EMD1_CMD_Command) -> AWR1_4/1(EMD1_CMD_Commamd)
  edcu_EMD1_CMD_SpeedRefLim/1 -> AWR1_4/3(EMD1_CMD_SpeedRefLim)
  pti_tqDesired_PTI1/1 -> AWR1_4/4(EMD1_CMD_TorqueRefLim)
  HVFreigabeHW1_SiRelay_D/1 -> AWR1_4/5(HVFreigabeHW_SiRelay_D)
  EMD1_CMD_Command1/1(Out_EMD1_CMD_Command) -> AWR1_4/14(EMD4_CMD_Commamd)
  edcu_EMD4_CMD_SpeedRefLim/1 -> AWR1_4/16(EMD4_CMD_SpeedRefLim)
  pti_tqDesired_PTI4/1 -> AWR1_4/17(EMD4_CMD_TorqueRefLim)
  HVFreigabeHW4_SiRelay_D/1 -> AWR1_4/18(HVFreigabeHW4_SiRelay_D)
  AWR1_4/1(awr1_4B) -> Bus Creator/2
  edcu_EMD2_CMD_ControlMode/1 -> EMD1_CMD_Command2/2(EMD1_CMD_MotorControlMode), AWR2_3/2(EMD2_CMD_MotorControlMode)
  edcu_EMD2_CMD_ClearErrors/1 -> EMD1_CMD_Command2/1(EMD1_CMD_ClearErrors)
  edcu_EMD3_CMD_ControlMode/1 -> EMD1_CMD_Command3/2(EMD1_CMD_MotorControlMode), AWR2_3/15(EMD3_CMD_MotorControlMode)
  edcu_EMD3_CMD_ClearErrors/1 -> EMD1_CMD_Command3/1(EMD1_CMD_ClearErrors)
  [TransInt] -> Unit Delay2/1
  Unit Delay2/1 -> Bus Selector3/1
  EMD1_CMD_Command2/1(Out_EMD1_CMD_Command) -> AWR2_3/1(EMD2_CMD_Commamd)
  edcu_EMD2_CMD_SpeedRefLim/1 -> AWR2_3/3(EMD2_CMD_SpeedRefLim)
  pti_tqDesired_PTI2/1 -> AWR2_3/4(EMD2_CMD_TorqueRefLim)
  HVFreigabeHW2_SiRelay_D/1 -> AWR2_3/5(HVFreigabeHW2_SiRelay_D)
  EMD1_CMD_Command3/1(Out_EMD1_CMD_Command) -> AWR2_3/14(EMD3_CMD_Commamd)
  edcu_EMD3_CMD_SpeedRefLim/1 -> AWR2_3/16(EMD3_CMD_SpeedRefLim)
  pti_tqDesired_PTI3/1 -> AWR2_3/17(EMD3_CMD_TorqueRefLim)
  HVFreigabeHW3_SiRelay_D/1 -> AWR2_3/18(HVFreigabeHW3_SiRelay_D)
  [vltZkBmsPhy] -> AWR2_3/6(vltZkBmsPhy)
  hvs_emot_Emot2_angVel/1 -> [hvs_emot_Emot2_angVel], AWR2_3/13(hvs_emot_Emot2_angVel)
  [hvs_emot_Emot1_angVel] -> Emot1_4/1(emot_Emot1_angVel)
  Bus Selector1/1 -> Emot1_4/3(trqEmotDesPhy1)  "<trqEmotDesPhy>"
  Bus Selector2/1 -> Emot1_4/5(trqEmotDesPhy4)  "<trqEmotDesPhy>"
  Emot1_4/1(emot1_4B) -> Bus Creator/3
  AWR2_3/1(awr2_3B) -> Bus Creator/1
  [TransInt] -> Bus Selector7/1
  [TransInt] -> Bus Selector8/1
  [hvs_emot_Emot2_angVel] -> Emot2_3/1(emot_Emot2_angVel)
  Bus Selector7/1 -> Emot2_3/3(trqEmotDesPhy2)  "<trqEmotDesPhy>"
  Bus Selector8/1 -> Emot2_3/5(trqEmotDesPhy3)  "<trqEmotDesPhy>"
  Emot2_3/1(emot2_3B) -> Bus Creator/4
  Bus Selector10/1 -> Bus Selector9/1, Bus Selector16/1  "TransInt"
  Bus Selector12/1 -> Bus Selector11/1, Bus Selector15/1  "TransInt"
  AWR 2 TX/1(hvs_EMD2_ACT_DigitalInput1) -> hvs_EMD2_ACT_DigitalInput1/1
  AWR 2 TX/2(hvs_EMD2_ACT_InverterState) -> hvs_EMD2_ACT_InverterState/1
  AWR 2 TX/3(hvs_EMD2_ACT_MaxAvailableTorque) -> hvs_EMD2_ACT_MaxAvailableTorque/1
  AWR 2 TX/4(hvs_EMD2_ACT_ReferenceTorqueLim) -> hvs_EMD2_ACT_ReferenceTorqueLim/1
  AWR 2 TX/5(hvs_EMD2_ACT_Torque) -> hvs_EMD2_ACT_Torque/1
  AWR 2 TX/6(hvs_EMD2_ACT_DcLinkPower) -> hvs_EMD2_ACT_DcLinkPower/1
  AWR 2 TX/7(hvs_EMD2_ACT_MotorSpeed) -> hvs_EMD2_ACT_MotorSpeed/1
  AWR 2 TX/8(hvs_EMD2_ACT_DcLinkVoltage) -> hvs_EMD2_ACT_DcLinkVoltage/1
  AWR 2 TX/17(hvs_EMD2_ACT_MaxJunctionTemp) -> hvs_EMD2_ACT_MaxJunctionTemp/1
  AWR 2 TX/9(hvs_EMD2_ACT_MotorTemperature) -> hvs_EMD2_ACT_MotorTemperature/1
  EDCU_Dig_SafetyCutOffDG1/1 -> [EDCU_Dig_SafetyCutOffDG1], AWR2_3/19(EDCU_Dig_SafetyCutOffDG1)
  [EDCU_Dig_SafetyCutOffDG1] -> AWR1_4/19(EDCU_Dig_SafetyCutOffDG1)
  SummarizeEmotorValuesForVehicle/2(hvs_emot_Emot2_torque) -> hvs_emot_Emot2_torque/1
  Bus Selector4/1 -> AWR1_4/9(pwEmot1Phy)  "<pwrEmotPhy>"
  Bus Selector4/2 -> AWR1_4/10(pwEmot4Phy)  "<pwrEmotPhy>"
  Bus Selector4/3 -> AWR1_4/11(trqEmot1Max)  "<trqEmotMax>"
  Bus Selector4/4 -> AWR1_4/12(trqEmot4Max)  "<trqEmotMax>"
  Bus Selector3/1 -> AWR2_3/9(pwEmot2Phy)  "<pwrEmotPhy>"
  Bus Selector3/2 -> AWR2_3/10(pwEmot3Phy)  "<pwrEmotPhy>"
  Bus Selector3/3 -> AWR2_3/11(trqEmot2Max)  "<trqEmotMax>"
  Bus Selector3/4 -> AWR2_3/12(trqEmot3Max)  "<trqEmotMax>"
  AWR 2 TX/11(hvs_EMD2_ACT_InverterLosses) -> hvs_EMD2_ACT_InverterLosses/1
  AWR 2 TX/12(hvs_EMD2_ACT_MotorLosses) -> hvs_EMD2_ACT_MotorLosses/1
  MotorSelection/1(Emot1_Selection) -> [Emot1_Selection]
  MotorSelection/2(Emot2_Selection) -> [Emot2_Selection]
  MotorSelection/3(Emot3_Selection) -> [Emot3_Selection]
  MotorSelection/4(Emot4_Selection) -> [Emot4_Selection]
  [Emot2_Selection] -> AWR2_3/20(Emot2_Selection)
  [Emot3_Selection] -> AWR2_3/21(Emot3_Selection)
  [Emot1_Selection] -> AWR1_4/20(Emot1_Selection)
  [Emot4_Selection] -> AWR1_4/21(Emot4_Selection)
  [Emot1_Selection] -> Emot1_4/15(Emot1_Selection)
  [Emot4_Selection] -> Emot1_4/16(Emot4_Selection)
  [Emot2_Selection] -> Emot2_3/15(Emot2_Selection)
  [Emot3_Selection] -> Emot2_3/16(Emot3_Selection)
  hvs_emot_Emot3_angVel/1 -> [hvs_emot_Emot3_angVel], AWR2_3/22(hvs_emot_Emot3_angVel)
  hvs_emot_Emot4_angVel/1 -> [hvs_emot_Emot4_angVel], AWR1_4/22(hvs_emot_Emot4_angVel)
  [hvs_emot_Emot4_angVel] -> Emot1_4/12(emot_Emot4_angVel)
  [hvs_emot_Emot3_angVel] -> Emot2_3/12(emot_Emot3_angVel)
  SummarizeEmotorValuesForVehicle/3(hvs_emot_Emot3_torque) -> hvs_emot_Emot3_torque/1
  SummarizeEmotorValuesForVehicle/4(hvs_emot_Emot4_torque) -> hvs_emot_Emot4_torque/1
  hvs_drvEmot4Oil_Temperature/1 -> Emot1_4/13(drvEmot4_Oil_Temperature)
  hvs_drvEmot2_Oil_Temperature/1 -> Emot2_3/6(drvEmot2_Oil_Temperature)
  hvs_drvEmot3Oil_Temperature/1 -> Emot2_3/13(drvEmot3_Oil_Temperature)
  SummarizeEmotorValuesForVehicle/8(hvs_drvEmot1WasteHeat_power) -> hvs_drvEmot1WasteHeat_power/1
  SummarizeEmotorValuesForVehicle/9(hvs_drvEmot2WasteHeat_power) -> hvs_drvEmot2WasteHeat_power/1
  SummarizeEmotorValuesForVehicle/10(hvs_drvEmot3WasteHeat_power) -> hvs_drvEmot3WasteHeat_power/1
  SummarizeEmotorValuesForVehicle/11(hvs_drvEmot4WasteHeat_power) -> hvs_drvEmot4WasteHeat_power/1
  hvs_drvEmot1_Coolant_Temperature/1 -> Emot1_4/7(drvEmot1_Coolant_Temperature)
  hvs_drvEmot_Ambient_Temperature/1 -> Emot2_3/8(drvEmot_Ambient_Temperature), Emot1_4/8(drvEmot_Ambient_Temperature)
  hvs_driveInverter1_switching_frequency/1 -> Emot1_4/10(inv1_switching_freq)
  hvs_drvEmot2_Coolant_Temperature/1 -> Emot2_3/7(drvEmot2_Coolant_Temperature)
  AWR 2 TX/10(hvs_EMD2_ACT_RotorTemperature) -> hvs_EMD2_ACT_RotorTemperature/1
  AWR 2 TX/13(hvs_EMD2_uStator) -> hvs_EMD2_uStator/1
  AWR 2 TX/14(hvs_EMD2_iStator) -> hvs_EMD2_iStator/1
  Bus Selector9/6 -> AWR 3 TX/6(IN_EMD3_ACT_Torque)  "<EMD_ACT_MotorTorque>"
  Bus Selector9/1 -> AWR 3 TX/1(IN_EMD3_ACT_DcLinkVoltage)  "<EMD3_ACT_DcLinkVoltage>"
  Bus Selector9/2 -> AWR 3 TX/2(IN_EMD3_ACT_DigitalInput1)  "<EMD_ACT_DigitalInput1>"
  Bus Selector9/4 -> AWR 3 TX/4(IN_EMD3_ACT_DcLinkPower)  "<EMD_ACT_DcLinkPower>"
  Bus Selector9/5 -> AWR 3 TX/5(IN_EMD3_ACT_MotorSpeed)  "<EMD_ACT_MotorSpeed>"
  Bus Selector9/7 -> AWR 3 TX/7(IN_EMD3_ACT_InverterState)  "<EMD_ACT_InverterState>"
  Bus Selector9/8 -> AWR 3 TX/8(IN_EMD3_ACT_ReferenceTorqueLimited)  "<EMD_ACT_ReferenceTorqueLimited>"
  Bus Selector9/3 -> AWR 3 TX/3(IN_EMD3_ACT_MaximumAvailableTorque)  "<EMD_ACT_MaximumAvailableTorque>"
  Bus Selector9/9 -> AWR 3 TX/9(IN_EMD3_ACT_MotorTemperature)  "<drvEmot_T_Stator>"
  Bus Selector9/10 -> AWR 3 TX/10(IN_EMD3_ACT_RotorTemperature)  "<drvEmot_T_Rotor>"
  Bus Selector9/12 -> AWR 3 TX/12(IN_EMD3_ACT_MotorLosses)  "<mot_Ploss>"
  Bus Selector9/13 -> AWR 3 TX/13(driveInverter_uStator)  "<uStator>"
  Bus Selector9/11 -> AWR 3 TX/11(IN_EMD3_ACT_InverterLosses)  "<Inv_Ploss>"
  Bus Selector9/14 -> AWR 3 TX/14(driveInverter_iStator)  "<iStator>"
  hvs_drvEmot4_Coolant_Temperature/1 -> Emot1_4/14(drvEmot4_Coolant_Temperature)
  hvs_drvEmot3_Coolant_Temperature/1 -> Emot2_3/14(drvEmot3_Coolant_Temperature)
  Bus Selector11/5 -> AWR 2 TX/5(IN_EMD2_ACT_MotorSpeed)  "<EMD_ACT_MotorSpeed>"
  Bus Selector11/6 -> AWR 2 TX/6(IN_EMD2_ACT_Torque)  "<EMD_ACT_MotorTorque>"
  Bus Selector11/2 -> AWR 2 TX/2(IN_EMD2_ACT_DigitalInput1)  "<EMD_ACT_DigitalInput1>"
  Bus Selector11/12 -> AWR 2 TX/12(IN_EMD2_ACT_MotorLosses)  "<mot_Ploss>"
  Bus Selector11/8 -> AWR 2 TX/8(IN_EMD2_ACT_ReferenceTorqueLimited)  "<EMD_ACT_ReferenceTorqueLimited>"
  Bus Selector11/9 -> AWR 2 TX/9(IN_EMD2_ACT_MotorTemperature)  "<drvEmot_T_Stator>"
  Bus Selector11/14 -> AWR 2 TX/14(driveInverter_iStator)  "<iStator>"
  Bus Selector11/3 -> AWR 2 TX/3(IN_EMD2_ACT_MaximumAvailableTorque)  "<EMD_ACT_MaximumAvailableTorque>"
  Bus Selector11/7 -> AWR 2 TX/7(IN_EMD2_ACT_InverterState)  "<EMD_ACT_InverterState>"
  Bus Selector11/4 -> AWR 2 TX/4(IN_EMD2_ACT_DcLinkPower)  "<EMD_ACT_DcLinkPower>"
  Bus Selector11/10 -> AWR 2 TX/10(IN_EMD2_ACT_RotorTemperature)  "<drvEmot_T_Rotor>"
  Bus Selector11/1 -> AWR 2 TX/1(IN_EMD2_ACT_DcLinkVoltage)  "<EMD2_ACT_DcLinkVoltage>"
  Bus Selector11/11 -> AWR 2 TX/11(IN_EMD2_ACT_InverterLosses)  "<Inv_Ploss>"
  Bus Selector11/13 -> AWR 2 TX/13(driveInverter_uStator)  "<uStator>"
  Bus Selector15/1 -> AWR 2 TX/17(driveInverter_Temperature_Bus)  "driveInverter_Temperatures_Bus"
  AWR 2 TX/18(hvs_EMD2_ACT_tSnsrPwrModlMax) -> hvs_EMD2_ACT_tSnsrPwrModlMax/1
  AWR 2 TX/19(hvs_EMD2_ACT_tCapSnsr) -> hvs_EMD2_ACT_tCapSnsr/1
  AWR 2 TX/20(hvs_EMD2_ACT_tCapCoil) -> hvs_EMD2_ACT_tCapCoil/1
  AWR 2 TX/21(hvs_EMD2_ACT_tCapAcCnctr) -> hvs_EMD2_ACT_tCapAcCnctr/1
  AWR 2 TX/22(hvs_EMD2_ACT_tCapDcCnctr) -> hvs_EMD2_ACT_tCapDcCnctr/1
  AWR 2 TX/23(hvs_EMD2_ACT_tIvtrAcRail) -> hvs_EMD2_ACT_tIvtrAcRail/1
  AWR 2 TX/24(hvs_EMD2_ACT_tIvtrDcRail) -> hvs_EMD2_ACT_tIvtrDcRail/1
  AWR 2 TX/25(hvs_EMD2_ACT_tIvtrAcRailIphaSnsr) -> hvs_EMD2_ACT_tIvtrAcRailIphaSnsr/1
  AWR 2 TX/26(hvs_EMD2_ACT_tIvtrDcRailCnctr) -> hvs_EMD2_ACT_tIvtrDcRailCnctr/1
  AWR 2 TX/27(hvs_EMD2_ACT_tCoolIvtrOuttk) -> hvs_EMD2_ACT_tCoolIvtrOuttk/1
  Bus Selector16/1 -> AWR 3 TX/17(driveInverter_Temperature_Bus)  "driveInverter_Temperatures_Bus"
  AWR 3 TX/1(hvs_EMD3_ACT_DigitalInput1) -> hvs_EMD3_ACT_DigitalInput1/1
  AWR 3 TX/2(hvs_EMD3_ACT_InverterState) -> hvs_EMD3_ACT_InverterState/1
  AWR 3 TX/3(hvs_EMD3_ACT_MaxAvailableTorque) -> hvs_EMD3_ACT_MaxAvailableTorque/1
  AWR 3 TX/4(hvs_EMD3_ACT_ReferenceTorqueLim) -> hvs_EMD3_ACT_ReferenceTorqueLim/1
  AWR 3 TX/5(hvs_EMD3_ACT_Torque) -> hvs_EMD3_ACT_Torque/1
  AWR 3 TX/6(hvs_EMD3_ACT_DcLinkPower) -> hvs_EMD3_ACT_DcLinkPower/1
  AWR 3 TX/7(hvs_EMD3_ACT_MotorSpeed) -> hvs_EMD3_ACT_MotorSpeed/1
  AWR 3 TX/8(hvs_EMD3_ACT_DcLinkVoltage) -> hvs_EMD3_ACT_DcLinkVoltage/1
  AWR 3 TX/9(hvs_EMD3_ACT_MotorTemperature) -> hvs_EMD3_ACT_MotorTemperature/1
  AWR 3 TX/10(hvs_EMD3_ACT_RotorTemperature) -> hvs_EMD3_ACT_RotorTemperature/1
  AWR 3 TX/11(hvs_EMD3_ACT_InverterLosses) -> hvs_EMD3_ACT_InverterLosses/1
  AWR 3 TX/12(hvs_EMD3_ACT_MotorLosses) -> hvs_EMD3_ACT_MotorLosses/1
  AWR 3 TX/13(hvs_EMD3_uStator) -> hvs_EMD3_uStator/1
  AWR 3 TX/14(hvs_EMD3_iStator) -> hvs_EMD3_iStator/1
  AWR 3 TX/17(hvs_EMD3_ACT_MaxJunctionTemp) -> hvs_EMD3_ACT_MaxJunctionTemp/1
  AWR 3 TX/18(hvs_EMD3_ACT_tSnsrPwrModlMax) -> hvs_EMD3_ACT_tSnsrPwrModlMax/1
  AWR 3 TX/19(hvs_EMD3_ACT_tCapSnsr) -> hvs_EMD3_ACT_tCapSnsr/1
  AWR 3 TX/20(hvs_EMD3_ACT_tCapCoil) -> hvs_EMD3_ACT_tCapCoil/1
  AWR 3 TX/21(hvs_EMD3_ACT_tCapAcCnctr) -> hvs_EMD3_ACT_tCapAcCnctr/1
  AWR 3 TX/22(hvs_EMD3_ACT_tCapDcCnctr) -> hvs_EMD3_ACT_tCapDcCnctr/1
  AWR 3 TX/23(hvs_EMD3_ACT_tIvtrAcRail) -> hvs_EMD3_ACT_tIvtrAcRail/1
  AWR 3 TX/24(hvs_EMD3_ACT_tIvtrDcRail) -> hvs_EMD3_ACT_tIvtrDcRail/1
  AWR 3 TX/25(hvs_EMD3_ACT_tIvtrAcRailIphaSnsr) -> hvs_EMD3_ACT_tIvtrAcRailIphaSnsr/1
  AWR 3 TX/26(hvs_EMD3_ACT_tIvtrDcRailCnctr) -> hvs_EMD3_ACT_tIvtrDcRailCnctr/1
  AWR 3 TX/27(hvs_EMD3_ACT_tCoolIvtrOuttk) -> hvs_EMD3_ACT_tCoolIvtrOuttk/1
  Bus Selector13/1 -> AWR 1 TX/1(IN_EMD1_ACT_DcLinkVoltage)  "<EMD1_ACT_DcLinkVoltage>"
  Bus Selector13/2 -> AWR 1 TX/2(IN_EMD1_ACT_DigitalInput1)  "<EMD_ACT_DigitalInput1>"
  Bus Selector13/3 -> AWR 1 TX/3(IN_EMD1_ACT_MaximumAvailableTorque)  "<EMD_ACT_MaximumAvailableTorque>"
  Bus Selector13/4 -> AWR 1 TX/4(IN_EMD1_ACT_DcLinkPower)  "<EMD_ACT_DcLinkPower>"
  Bus Selector13/5 -> AWR 1 TX/5(IN_EMD1_ACT_MotorSpeed)  "<EMD_ACT_MotorSpeed>"
  Bus Selector13/6 -> AWR 1 TX/6(IN_EMD1_ACT_Torque)  "<EMD_ACT_MotorTorque>"
  Bus Selector13/7 -> AWR 1 TX/7(IN_EMD1_ACT_InverterState)  "<EMD_ACT_InverterState>"
  Bus Selector13/8 -> AWR 1 TX/8(IN_EMD1_ACT_ReferenceTorqueLimited)  "<EMD_ACT_ReferenceTorqueLimited>"
  Bus Selector13/9 -> AWR 1 TX/9(IN_EMD1_ACT_MotorTemperature)  "<drvEmot_T_Stator>"
  Bus Selector13/10 -> AWR 1 TX/10(IN_EMD1_ACT_RotorTemperature)  "<drvEmot_T_Rotor>"
  Bus Selector13/11 -> AWR 1 TX/11(IN_EMD1_ACT_InverterLosses)  "<Inv_Ploss>"
  Bus Selector13/12 -> AWR 1 TX/12(IN_EMD1_ACT_MotorLosses)  "<mot_Ploss>"
  Bus Selector13/13 -> AWR 1 TX/13(driveInverter_uStator)  "<uStator>"
  Bus Selector13/14 -> AWR 1 TX/14(driveInverter_iStator)  "<iStator>"
  Bus Selector17/1 -> AWR 1 TX/17(driveInverter_Temperature_Bus)  "driveInverter_Temperatures_Bus"
  AWR 1 TX/1(hvs_EMD1_ACT_DigitalInput1) -> hvs_EMD1_ACT_DigitalInput1/1
  AWR 1 TX/2(hvs_EMD1_ACT_InverterState) -> hvs_EMD1_ACT_InverterState/1
  AWR 1 TX/3(hvs_EMD1_ACT_MaxAvailableTorque) -> hvs_EMD1_ACT_MaxAvailableTorque/1
  AWR 1 TX/4(hvs_EMD1_ACT_ReferenceTorqueLim) -> hvs_EMD1_ACT_ReferenceTorqueLim/1
  AWR 1 TX/5(hvs_EMD1_ACT_Torque) -> hvs_EMD1_ACT_Torque/1
  AWR 1 TX/6(hvs_EMD1_ACT_DcLinkPower) -> hvs_EMD1_ACT_DcLinkPower/1
  AWR 1 TX/7(hvs_EMD1_ACT_MotorSpeed) -> hvs_EMD1_ACT_MotorSpeed/1
  AWR 1 TX/8(hvs_EMD1_ACT_DcLinkVoltage) -> hvs_EMD1_ACT_DcLinkVoltage/1
  AWR 1 TX/9(hvs_EMD1_ACT_MotorTemperature) -> hvs_EMD1_ACT_MotorTemperature/1
  AWR 1 TX/10(hvs_EMD1_ACT_RotorTemperature) -> hvs_EMD1_ACT_RotorTemperature/1
  AWR 1 TX/11(hvs_EMD1_ACT_InverterLosses) -> hvs_EMD1_ACT_InverterLosses/1
  AWR 1 TX/12(hvs_EMD1_ACT_MotorLosses) -> hvs_EMD1_ACT_MotorLosses/1
  AWR 1 TX/13(hvs_EMD1_uStator) -> hvs_EMD1_uStator/1
  AWR 1 TX/14(hvs_EMD1_iStator) -> hvs_EMD1_iStator/1
  AWR 1 TX/17(hvs_EMD1_ACT_MaxJunctionTemp) -> hvs_EMD1_ACT_MaxJunctionTemp/1
  AWR 1 TX/18(hvs_EMD1_ACT_tSnsrPwrModlMax) -> hvs_EMD1_ACT_tSnsrPwrModlMax/1
  AWR 1 TX/19(hvs_EMD1_ACT_tCapSnsr) -> hvs_EMD1_ACT_tCapSnsr/1
  AWR 1 TX/20(hvs_EMD1_ACT_tCapCoil) -> hvs_EMD1_ACT_tCapCoil/1
  AWR 1 TX/21(hvs_EMD1_ACT_tCapAcCnctr) -> hvs_EMD1_ACT_tCapAcCnctr/1
  AWR 1 TX/22(hvs_EMD1_ACT_tCapDcCnctr) -> hvs_EMD1_ACT_tCapDcCnctr/1
  AWR 1 TX/23(hvs_EMD1_ACT_tIvtrAcRail) -> hvs_EMD1_ACT_tIvtrAcRail/1
  AWR 1 TX/24(hvs_EMD1_ACT_tIvtrDcRail) -> hvs_EMD1_ACT_tIvtrDcRail/1
  AWR 1 TX/25(hvs_EMD1_ACT_tIvtrAcRailIphaSnsr) -> hvs_EMD1_ACT_tIvtrAcRailIphaSnsr/1
  AWR 1 TX/26(hvs_EMD1_ACT_tIvtrDcRailCnctr) -> hvs_EMD1_ACT_tIvtrDcRailCnctr/1
  AWR 1 TX/27(hvs_EMD1_ACT_tCoolIvtrOuttk) -> hvs_EMD1_ACT_tCoolIvtrOuttk/1
  Bus Selector14/1 -> AWR 4 TX/1(IN_EMD4_ACT_DcLinkVoltage)  "<EMD4_ACT_DcLinkVoltage>"
  Bus Selector14/2 -> AWR 4 TX/2(IN_EMD4_ACT_DigitalInput1)  "<EMD_ACT_DigitalInput1>"
  Bus Selector14/3 -> AWR 4 TX/3(IN_EMD4_ACT_MaximumAvailableTorque)  "<EMD_ACT_MaximumAvailableTorque>"
  Bus Selector14/4 -> AWR 4 TX/4(IN_EMD4_ACT_DcLinkPower)  "<EMD_ACT_DcLinkPower>"
  Bus Selector14/5 -> AWR 4 TX/5(IN_EMD4_ACT_MotorSpeed)  "<EMD_ACT_MotorSpeed>"
  Bus Selector14/6 -> AWR 4 TX/6(IN_EMD4_ACT_Torque)  "<EMD_ACT_MotorTorque>"
  Bus Selector14/7 -> AWR 4 TX/7(IN_EMD4_ACT_InverterState)  "<EMD_ACT_InverterState>"
  Bus Selector14/8 -> AWR 4 TX/8(IN_EMD4_ACT_ReferenceTorqueLimited)  "<EMD_ACT_ReferenceTorqueLimited>"
  Bus Selector14/9 -> AWR 4 TX/9(IN_EMD4_ACT_MotorTemperature)  "<drvEmot_T_Stator>"
  Bus Selector14/10 -> AWR 4 TX/10(IN_EMD4_ACT_RotorTemperature)  "<drvEmot_T_Rotor>"
  Bus Selector14/11 -> AWR 4 TX/11(IN_EMD4_ACT_InverterLosses)  "<Inv_Ploss>"
  Bus Selector14/12 -> AWR 4 TX/12(IN_EMD4_ACT_MotorLosses)  "<mot_Ploss>"
  Bus Selector14/13 -> AWR 4 TX/13(driveInverter_uStator)  "<uStator>"
  Bus Selector14/14 -> AWR 4 TX/14(driveInverter_iStator)  "<iStator>"
  Bus Selector18/1 -> AWR 4 TX/17(driveInverter_Temperature_Bus)  "driveInverter_Temperatures_Bus"
  AWR 4 TX/1(hvs_EMD4_ACT_DigitalInput1) -> hvs_EMD4_ACT_DigitalInput1/1
  AWR 4 TX/2(hvs_EMD4_ACT_InverterState) -> hvs_EMD4_ACT_InverterState/1
  AWR 4 TX/3(hvs_EMD4_ACT_MaxAvailableTorque) -> hvs_EMD4_ACT_MaxAvailableTorque/1
  AWR 4 TX/4(hvs_EMD4_ACT_ReferenceTorqueLim) -> hvs_EMD4_ACT_ReferenceTorqueLim/1
  AWR 4 TX/5(hvs_EMD4_ACT_Torque) -> hvs_EMD4_ACT_Torque/1
  AWR 4 TX/6(hvs_EMD4_ACT_DcLinkPower) -> hvs_EMD4_ACT_DcLinkPower/1
  AWR 4 TX/7(hvs_EMD4_ACT_MotorSpeed) -> hvs_EMD4_ACT_MotorSpeed/1
  AWR 4 TX/8(hvs_EMD4_ACT_DcLinkVoltage) -> hvs_EMD4_ACT_DcLinkVoltage/1
  AWR 4 TX/9(hvs_EMD4_ACT_MotorTemperature) -> hvs_EMD4_ACT_MotorTemperature/1
  AWR 4 TX/10(hvs_EMD4_ACT_RotorTemperature) -> hvs_EMD4_ACT_RotorTemperature/1
  AWR 4 TX/11(hvs_EMD4_ACT_InverterLosses) -> hvs_EMD4_ACT_InverterLosses/1
  AWR 4 TX/12(hvs_EMD4_ACT_MotorLosses) -> hvs_EMD4_ACT_MotorLosses/1
  AWR 4 TX/13(hvs_EMD4_uStator) -> hvs_EMD4_uStator/1
  AWR 4 TX/14(hvs_EMD4_iStator) -> hvs_EMD4_iStator/1
  AWR 4 TX/17(hvs_EMD4_ACT_MaxJunctionTemp) -> hvs_EMD4_ACT_MaxJunctionTemperature/1
  AWR 4 TX/18(hvs_EMD4_ACT_tSnsrPwrModlMax) -> hvs_EMD4_ACT_tSnsrPwrModlMax/1
  AWR 4 TX/19(hvs_EMD4_ACT_tCapSnsr) -> hvs_EMD4_ACT_tCapSnsr/1
  AWR 4 TX/20(hvs_EMD4_ACT_tCapCoil) -> hvs_EMD4_ACT_tCapCoil/1
  AWR 4 TX/21(hvs_EMD4_ACT_tCapAcCnctr) -> hvs_EMD4_ACT_tCapAcCnctr/1
  AWR 4 TX/22(hvs_EMD4_ACT_tCapDcCnctr) -> hvs_EMD4_ACT_tCapDcCnctr/1
  AWR 4 TX/23(hvs_EMD4_ACT_tIvtrAcRail) -> hvs_EMD4_ACT_tIvtrAcRail/1
  AWR 4 TX/24(hvs_EMD4_ACT_tIvtrDcRail) -> hvs_EMD4_ACT_tIvtrDcRail/1
  AWR 4 TX/25(hvs_EMD4_ACT_tIvtrAcRailIphaSnsr) -> hvs_EMD4_ACT_tIvtrAcRailIphaSnsr/1
  AWR 4 TX/26(hvs_EMD4_ACT_tIvtrDcRailCnctr) -> hvs_EMD4_ACT_tIvtrDcRailCnctr/1
  AWR 4 TX/27(hvs_EMD4_ACT_tCoolIvtrOuttk) -> hvs_EMD4_ACT_tCoolIvtrOuttk/1
  Bus Selector11/15 -> AWR 2 TX/15(driveInverter_modIdx)  "<modIdx>"
  Bus Selector11/16 -> AWR 2 TX/16(driveInverter_cosPhi)  "<cosPhi>"
  AWR 2 TX/15(hvs_EMD2_modIdx) -> hvs_EMD2_modIdx/1
  AWR 2 TX/16(hvs_EMD2_cosPhi) -> hvs_EMD2_cosPhi/1
  Bus Selector14/15 -> AWR 4 TX/15(driveInverter_modIdx)  "<modIdx>"
  Bus Selector14/16 -> AWR 4 TX/16(driveInverter_cosPhi)  "<cosPhi>"
  AWR 4 TX/16(hvs_EMD4_cosPhi) -> hvs_EMD4_cosPhi/1
  AWR 4 TX/15(hvs_EMD4_modIdx) -> hvs_EMD4_modIdx/1
  AWR 1 TX/15(hvs_EMD1_modIdx) -> hvs_EMD1_modIdx/1
  AWR 1 TX/16(hvs_EMD1_cosPhi) -> hvs_EMD1_cosPhi/1
  Bus Selector13/15 -> AWR 1 TX/15(driveInverter_modIdx)  "<modIdx>"
  Bus Selector13/16 -> AWR 1 TX/16(driveInverter_cosPhi)  "<cosPhi>"
  AWR 3 TX/15(hvs_EMD3_modIdx) -> hvs_EMD3_modIdx/1
  AWR 3 TX/16(hvs_EMD3_cosPhi) -> hvs_EMD3_cosPhi/1
  Bus Selector9/15 -> AWR 3 TX/15(driveInverter_modIdx)  "<modIdx>"
  Bus Selector9/16 -> AWR 3 TX/16(driveInverter_cosPhi)  "<cosPhi>"
  hvs_driveInverter4_switching_frequency/1 -> Emot1_4/11(inv4_switching_freq)
  hvs_driveInverter3_switching_frequency/1 -> Emot2_3/11(inv3_switching_freq)
  hvs_driveInverter2_switching_frequency/1 -> Emot2_3/10(inv2_switching_freq)
  hvs_drvEmot1CoolantFlow_vdot/1 -> Emot1_4/17(drvEmot1CoolantFlow_vdot)
  hvs_drvEmot1OilFlow_vdot/1 -> Emot1_4/18(drvEmot1OilFlow_vdot)
  hvs_driveInverterCoolantFlow_vdot/1 -> Emot2_3/19(driveInverterCoolantFlow_vdot), Emot1_4/19(driveInverterCoolantFlow_vdot)
  hvs_drvEmot4CoolantFlow_vdot/1 -> Emot1_4/20(drvEmot4CoolantFlow_vdot)
  hvs_drvEmot4OilFlow_vdot/1 -> Emot1_4/21(drvEmot4OilFlow_vdot)
  hvs_drvEmot3OilFlow_vdot/1 -> Emot2_3/21(drvEmot3OilFlow_vdot)
  hvs_drvEmot2CoolantFlow_vdot/1 -> Emot2_3/17(drvEmot2CoolantFlow_vdot)
  hvs_drvEmot3CoolantFlow_vdot/1 -> Emot2_3/20(drvEmot3CoolantFlow_vdot)
  hvs_drvEmot2OilFlow_vdot/1 -> Emot2_3/18(drvEmot2OilFlow_vdot)
  Unit Delay1/1 -> Bus Selector20/1
  Unit Delay4/1 -> Bus Selector19/1
  AWR 2 TX/28(hvs_EMD2_ACT_Torque_Nm) -> hvs_EMD2_ACT_Torque_Nm/1
  AWR 3 TX/28(hvs_EMD3_ACT_Torque_Nm) -> hvs_EMD3_ACT_Torque_Nm/1
  AWR 1 TX/28(hvs_EMD1_ACT_Torque_Nm) -> hvs_EMD1_ACT_Torque_Nm/1
  AWR 4 TX/28(hvs_EMD4_ACT_Torque_Nm) -> hvs_EMD4_ACT_Torque_Nm/1
  Bus Selector11/17 -> AWR 2 TX/18(IN_drvEmot2WasteHeatcoolant_power)  "<wasteHeat_coolant>"
  Bus Selector11/18 -> AWR 2 TX/19(IN_drvEmot2WasteHeatoil_power)  "<wasteHeat_oil>"
  Bus Selector9/17 -> AWR 3 TX/18(IN_drvEmot3WasteHeatcoolant_power)  "<wasteHeat_oil>"
  Bus Selector9/18 -> AWR 3 TX/19(IN_drvEmot3WasteHeatoil_power)  "<wasteHeat_coolant>"
  Bus Selector13/17 -> AWR 1 TX/18(IN_drvEmot1WasteHeatcoolant_power)  "<wasteHeat_coolant>"
  Bus Selector13/18 -> AWR 1 TX/19(IN_drvEmot1WasteHeatoil_power)  "<wasteHeat_oil>"
  Bus Selector14/17 -> AWR 4 TX/18(IN_drvEmot4WasteHeatcoolant_power)  "<wasteHeat_coolant>"
  Bus Selector14/18 -> AWR 4 TX/19(IN_drvEmot4WasteHeatoil_power)  "<wasteHeat_oil>"
  AWR 2 TX/30(hvs_drvEmot2WasteHeatoil_power) -> hvs_drvEmot2WasteHeatoil_power/1
  AWR 2 TX/29(hvs_drvEmot2WasteHeatcoolant_power) -> hvs_drvEmot2WasteHeatcoolant_power/1
  AWR 3 TX/30(hvs_drvEmot3WasteHeatoil_power) -> hvs_drvEmot3WasteHeatoil_power/1
  AWR 3 TX/29(hvs_drvEmot3WasteHeatcoolant_power) -> hvs_drvEmot3WasteHeatcoolant_power/1
  AWR 1 TX/29(hvs_drvEmot1WasteHeatcoolant_power) -> hvs_drvEmot1WasteHeatcoolant_power/1
  AWR 1 TX/30(hvs_drvEmot1WasteHeatoil_power) -> hvs_drvEmot1WasteHeatoil_power/1
  AWR 4 TX/29(hvs_drvEmot4WasteHeatcoolant_power) -> hvs_drvEmot4WasteHeatcoolant_power/1
  AWR 4 TX/30(hvs_drvEmot4WasteHeatoil_power) -> hvs_drvEmot4WasteHeatoil_power/1
  [vltZkBmsPhy] -> Emot1_4/4(voltBatHV4), Emot1_4/2(voltBatHV1)
  [vltZkBmsPhy] -> Emot2_3/4(voltBatHV3), Emot2_3/2(voltBatHV2)
